simulink model "power_demand"  (R2023a)
settings: Solver=VariableStepAuto  StartTime=0.0  StopTime=1800  RelTol=1e-3
values from neighbouring files (symbols this model uses):
  sim_case = i    [create_SOC_dataset.m]    (also in create_csv.m = 2; setHESSParam.m = 6; setHESSParamv2.m = 6)
libraries: autolibshared x1
settings Model: Creator=tu101  LastModifiedBy=tu101

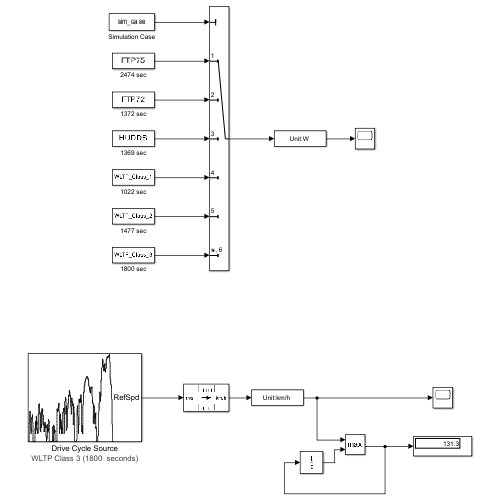
[thumbnail: Simulink's stored preview of the top-level diagram]
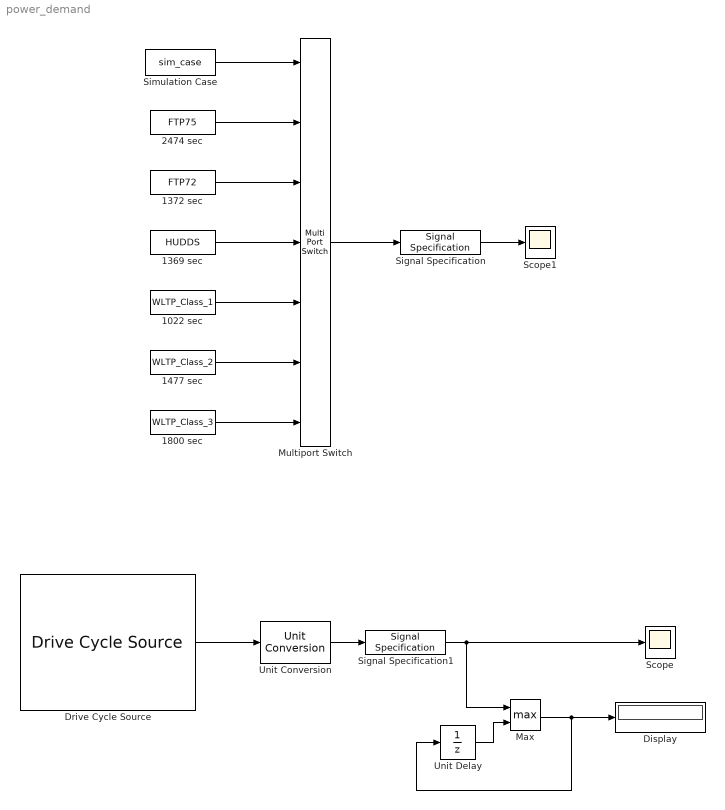
== system power_demand ==
  1022 sec : FromWorkspace  VariableName=WLTP_Class_1  Interpolate=off  ZeroCross=off  OutputAfterFinalValue=Setting to zero
  1369 sec : FromWorkspace  VariableName=HUDDS  Interpolate=off  ZeroCross=off  OutputAfterFinalValue=Setting to zero
  1372 sec : FromWorkspace  VariableName=FTP72  Interpolate=off  ZeroCross=off  OutputAfterFinalValue=Setting to zero
  1477 sec : FromWorkspace  VariableName=WLTP_Class_2  Interpolate=off  ZeroCross=off  OutputAfterFinalValue=Setting to zero
  1800 sec : FromWorkspace  VariableName=WLTP_Class_3  Interpolate=off  ZeroCross=off  OutputAfterFinalValue=Setting to zero
  2474 sec : FromWorkspace  VariableName=FTP75  Interpolate=off  ZeroCross=off  OutputAfterFinalValue=Setting to zero
  Display : Display
  Drive Cycle Source : autolibshared/Drive Cycle Source  cycleVar=WLTP Class 3  fileVar=cycleFTP75.mat  tfinal="1800  seconds"  cycleRepeat=off  outAccPort=off  outGearPort=off  gearList=No gear data  t_wot1=5  xdot_woto=0  xdot_wot1=30  t_wot2=20  xdot_wot2=0  t_wotend=30  srcUnit=m/s  outUnit=m/s  srcAccUnit=m/s/s  outAccUnit=m/s^2  dt=0  aMode=1  faultOption=off  velBnd=2  velBndUnit=mph  inUnit=m/s  timeBnd=1  failOption=off  stopSim=off  maxFaultCnt=10  maxFaultTime=2  maxTotFaultTime=15  traceOption=off  dtTrace=1  traceWindow=10  lastDCname=Artemis Rural Road  lastOutUnit=mph  lastDT=0  lastTB=1  lastSB=2  forceCalcBound=off
  Max : MinMax  Function=max  Inputs=2
  Multiport Switch : MultiPortSwitch  Inputs=6  SaturateOnIntegerOverflow=off  InputSameDT=off
  Scope : Scope
  Scope1 : Scope
  Signal Specification : SignalSpecification  Unit=W
  Signal Specification1 : SignalSpecification  Unit=km/h
  Simulation Case : Constant  Value=sim_case
  Unit Conversion : UnitConversion
  Unit Delay : UnitDelay  SampleTime=-1  HasFrameUpgradeWarning=on
  wires:
  Unit Delay/1 -> Max/2
  Signal Specification1/1 -> Max/1, Scope/1
  1477 sec/1 -> Multiport Switch/6
  Drive Cycle Source/1 -> Unit Conversion/1
  Max/1 -> Display/1, Unit Delay/1
  Simulation Case/1 -> Multiport Switch/1
  1022 sec/1 -> Multiport Switch/5
  2474 sec/1 -> Multiport Switch/2
  1372 sec/1 -> Multiport Switch/3
  Multiport Switch/1 -> Signal Specification/1
  1369 sec/1 -> Multiport Switch/4
  Signal Specification/1 -> Scope1/1
  1800 sec/1 -> Multiport Switch/7
  Unit Conversion/1 -> Signal Specification1/1
